simulink model "LCK_DanishV01"  (R2018b)
settings: Solver=FixedStepDiscrete  StartTime=0.0  StopTime=inf  FixedStep=0.01  RelTol=1e-3
PostLoadFcn:
  | if any(exist('dsrtsu_mdlpostloadfcn', 'file') ~= 0), dsrtsu_mdlpostloadfcn('Execute', bdroot); end
values from neighbouring files (symbols this model uses):
  C_DEG2RAD = 0.0175    [LCK_Macro.sldd]
  C_KPH2MPS = 0.2778    [LCK_Macro.sldd]
  C_NEARZERO = 0.0001    [LCK_Macro.sldd]
  C_ONE = 1.0    [LCK_Macro.sldd]
  C_RAD2DEG = 57.2958    [LCK_Macro.sldd]
  C_ZERO = 0.0    [LCK_Macro.sldd]
  k_accel_pedal_pos_per_speed_x : value not decoded    [LCK_LogicPara.sldd]
  k_accel_pedal_pos_per_speed_z : value not decoded    [LCK_LogicPara.sldd]
  k_brake_suprress_hold = 1000.0    [LCK_LogicPara.sldd]
  k_driver_appl_torque_filt = 50.0    [LCK_LogicPara.sldd]
  k_driver_suppression_hold_time = 3000.0    [LCK_LogicPara.sldd]
  k_hands_on_wheel_hold_msec = 500.0    [LCK_LogicPara.sldd]
  k_hands_on_wheel_torque_hi = 0.2    [LCK_LogicPara.sldd]
  k_hands_on_wheel_torque_lo = 0.15    [LCK_LogicPara.sldd]
  k_handsoff_delay_cycles = 50.0    [LCK_LogicPara.sldd]
  k_handsoff_torq_Lo_CR = 0.3    [LCK_LogicPara.sldd]
  k_handson_delay_cycles = 5.0    [LCK_LogicPara.sldd]
  k_HighAccel_suppress_hold = 3000.0    [LCK_LogicPara.sldd]
  k_HLR_suprress_hold = 3000.0    [LCK_LogicPara.sldd]
  k_hs_StrAng_CR_threshold_z : value not decoded    [LCK_LogicPara.sldd]
  k_LC_Exit_Switch = 0.0    [LCK_LogicPara.sldd]
  k_LCG_Configured = 1.0    [LCK_LogicPara.sldd]
  k_LCK_A0_Rdy2Act_UseConst = 0.0    [LCK_LogicPara.sldd]
  k_LCK_A0Fac_ActSta : value not decoded    [LCK_CtrlPara.sldd]
  k_LCK_A0Fac_DrvStm : value not decoded    [LCK_CtrlPara.sldd]
  k_LCK_A0Shift_LftCurv : value not decoded    [LCK_CtrlPara.sldd]
  k_LCK_A0Shift_RgtCurv : value not decoded    [LCK_CtrlPara.sldd]
  k_LCK_A0Shift_StraLan = 0.0    [LCK_CtrlPara.sldd]
  k_LCK_A0ShiftFac_Dy_LftCurv : value not decoded    [LCK_CtrlPara.sldd]
  k_LCK_A0ShiftFac_Dy_RgtCurv : value not decoded    [LCK_CtrlPara.sldd]
  k_LCK_A0ShiftFac_Vspd : value not decoded    [LCK_CtrlPara.sldd]
  k_LCK_accel_inhibit_thold = 35.0    [LCK_LogicPara.sldd]
  k_LCK_Active2Ready_Mask = 255.0    [LCK_LogicPara.sldd]
  k_LCK_CvatRateBks : value not decoded    [LCK_CtrlPara.sldd]
  k_LCK_CvatrBks : value not decoded    [LCK_CtrlPara.sldd]
  k_LCK_DFac_Dy : value not decoded    [LCK_CtrlPara.sldd]
  k_LCK_DFac_Dy_Curv : value not decoded    [LCK_CtrlPara.sldd]
  k_LCK_DFac_HaCurCen : value not decoded    [LCK_CtrlPara.sldd]
  k_LCK_DFac_HaCurSid : value not decoded    [LCK_CtrlPara.sldd]
  k_LCK_DFac_HadCurCen : value not decoded    [LCK_CtrlPara.sldd]
  k_LCK_DFac_HadCurSid : value not decoded    [LCK_CtrlPara.sldd]
  k_LCK_DFac_HadStrCen : value not decoded    [LCK_CtrlPara.sldd]
  k_LCK_DFac_HadStrSid : value not decoded    [LCK_CtrlPara.sldd]
  k_LCK_DFac_HaStrCen : value not decoded    [LCK_CtrlPara.sldd]
  k_LCK_DFac_HaStrSid : value not decoded    [LCK_CtrlPara.sldd]
  k_LCK_DFac_Rad : value not decoded    [LCK_CtrlPara.sldd]
  k_LCK_DFac_SA_CurCen : value not decoded    [LCK_CtrlPara.sldd]
  k_LCK_DFac_SA_CurSid : value not decoded    [LCK_CtrlPara.sldd]
  k_LCK_DFac_SA_StrCen : value not decoded    [LCK_CtrlPara.sldd]
  k_LCK_DFac_SA_StrSid : value not decoded    [LCK_CtrlPara.sldd]
  k_LCK_DFac_SS_CurCen : value not decoded    [LCK_CtrlPara.sldd]
  k_LCK_DFac_SS_CurSid : value not decoded    [LCK_CtrlPara.sldd]
  k_LCK_DFac_SS_StrCen : value not decoded    [LCK_CtrlPara.sldd]
  k_LCK_DFac_SS_StrSid : value not decoded    [LCK_CtrlPara.sldd]
  k_LCK_DFac_Vspd : value not decoded    [LCK_CtrlPara.sldd]
  k_LCK_DlyTm_DrvStim = 0.2    [LCK_CtrlPara.sldd]
  k_LCK_DTermMax = 2.0    [LCK_CtrlPara.sldd]
  k_LCK_DyBks_Curv : value not decoded    [LCK_CtrlPara.sldd]
  k_LCK_Enable_POOnly = 1.0    [LCK_LogicPara.sldd]
  k_LCK_Entry_DistBuffer = 0.1    [LCK_LogicPara.sldd]
  k_LCK_Fac_Vspd2RngThr_FalRec = 0.23    [LCK_CtrlPara.sldd]
  k_LCK_Ffw_CvatSwh = 0.0    [LCK_CtrlPara.sldd]
  k_LCK_Ffw_DyBks : value not decoded    [LCK_CtrlPara.sldd]
  k_LCK_Ffw_TimCon_CmdFlt = 0.0    [LCK_CtrlPara.sldd]
  k_LCK_FfwDeltaFac_Rad_Lft : value not decoded    [LCK_CtrlPara.sldd]
  k_LCK_FfwDeltaFac_Rad_Rgt : value not decoded    [LCK_CtrlPara.sldd]
  k_LCK_FfwDeltaFac_Vspd : value not decoded    [LCK_CtrlPara.sldd]
  k_LCK_FfwFac_CvatRate_Lft : value not decoded    [LCK_CtrlPara.sldd]
  k_LCK_FfwFac_CvatRate_Rgt : value not decoded    [LCK_CtrlPara.sldd]
  k_LCK_FfwFac_Dy : value not decoded    [LCK_CtrlPara.sldd]
  k_LCK_FfwFac_Rad_Lft : value not decoded    [LCK_CtrlPara.sldd]
  k_LCK_FfwFac_Rad_Rgt : value not decoded    [LCK_CtrlPara.sldd]
  k_LCK_FfwFac_Vspd : value not decoded    [LCK_CtrlPara.sldd]
  k_LCK_FfwTorq_Cvat : value not decoded    [LCK_CtrlPara.sldd]
  k_LCK_HAFac_ActSta : value not decoded    [LCK_CtrlPara.sldd]
  k_LCK_HAFac_DrvStm : value not decoded    [LCK_CtrlPara.sldd]
  k_LCK_HaloTime = 2000.0    [LCK_LogicPara.sldd]
  k_LCK_HaloTime_Switch = 0.0    [LCK_LogicPara.sldd]
  k_LCK_HARFac_ActSta : value not decoded    [LCK_CtrlPara.sldd]
  k_LCK_HARFac_DrvStm : value not decoded    [LCK_CtrlPara.sldd]
  k_LCK_Hed_DyBks : value not decoded    [LCK_CtrlPara.sldd]
  k_LCK_HedAngDiffX : value not decoded    [LCK_CtrlPara.sldd]
  k_LCK_HedAngRateDiffX : value not decoded    [LCK_CtrlPara.sldd]
  k_LCK_HndsOnWhel_DlyTm_Idl2Rdy = 0.0    [LCK_LogicPara.sldd]
  k_LCK_host_veh_width = 1.86    [LCK_LogicPara.sldd]
  k_LCK_Idle2Ready_Mask = 239.0    [LCK_LogicPara.sldd]
  k_LCK_Junc_SusTime = 1.0    [LCK_LogicPara.sldd]
  k_LCK_KpKdDecSlopeLmt = 10.0    [LCK_CtrlPara.sldd]
  k_LCK_KpKdIncSlopeLmt = 5.0    [LCK_CtrlPara.sldd]
  k_LCK_Lat_Ctrl_DFac_Lft = 1.0    [LCK_CtrlPara.sldd]
  k_LCK_Lat_Ctrl_DFac_Rgt = 1.05    [LCK_CtrlPara.sldd]
  k_LCK_Lat_Ctrl_Kd = 0.8    [LCK_CtrlPara.sldd]
  k_LCK_Lat_Ctrl_Ki = 0.5    [LCK_CtrlPara.sldd]
  k_LCK_Lat_Ctrl_Kp = 0.7    [LCK_CtrlPara.sldd]
  k_LCK_Lat_Ctrl_Kp_NearGain = 0.7    [LCK_CtrlPara.sldd]
  k_LCK_Lat_Ctrl_PFac_Lft = 1.0    [LCK_CtrlPara.sldd]
  k_LCK_Lat_Ctrl_PFac_Rgt = 1.05    [LCK_CtrlPara.sldd]
  k_LCK_Lat_Ctrl_TimCon_CmdFlt = 5.0    [LCK_CtrlPara.sldd]
  k_LCK_Lat_DFac_Rad : value not decoded    [LCK_CtrlPara.sldd]
  k_LCK_Lat_DFac_SS_Cur : value not decoded    [LCK_CtrlPara.sldd]
  k_LCK_Lat_DFac_SS_Str : value not decoded    [LCK_CtrlPara.sldd]
  k_LCK_Lat_DFac_Vspd : value not decoded    [LCK_CtrlPara.sldd]
  k_LCK_Lat_DyBks : value not decoded    [LCK_CtrlPara.sldd]
  k_LCK_Lat_IFac_Rad : value not decoded    [LCK_CtrlPara.sldd]
  k_LCK_Lat_IFac_Vspd : value not decoded    [LCK_CtrlPara.sldd]
  k_LCK_Lat_ILmtFac_Dy_CurvLan : value not decoded    [LCK_CtrlPara.sldd]
  k_LCK_Lat_ILmtFac_Dy_StraLan : value not decoded    [LCK_CtrlPara.sldd]
  k_LCK_Lat_ILmtFac_Rad : value not decoded    [LCK_CtrlPara.sldd]
  k_LCK_Lat_ILmtFac_Rad_NearGain = 1.0    [LCK_CtrlPara.sldd]
  k_LCK_Lat_ILmtFac_Vspd_CurvLan : value not decoded    [LCK_CtrlPara.sldd]
  k_LCK_Lat_ILmtFac_Vspd_StraLan : value not decoded    [LCK_CtrlPara.sldd]
  k_LCK_Lat_ITermLmt_Dy = 1.0    [LCK_CtrlPara.sldd]
  k_LCK_Lat_KpKdDecSlopeLmt = 10.0    [LCK_CtrlPara.sldd]
  k_LCK_Lat_KpKdIncSlopeLmt = 10.0    [LCK_CtrlPara.sldd]
  k_LCK_Lat_PFac_Dy_InnLftCur : value not decoded    [LCK_CtrlPara.sldd]
  k_LCK_Lat_PFac_Dy_InnRgtCur : value not decoded    [LCK_CtrlPara.sldd]
  k_LCK_Lat_PFac_Dy_OutLftCur : value not decoded    [LCK_CtrlPara.sldd]
  k_LCK_Lat_PFac_Dy_OutRgtCur : value not decoded    [LCK_CtrlPara.sldd]
  k_LCK_Lat_PFac_Dy_Str : value not decoded    [LCK_CtrlPara.sldd]
  k_LCK_Lat_PFac_Rad : value not decoded    [LCK_CtrlPara.sldd]
  ... (+153 more)
undefined symbols (not defined in the file or in its folder): k_LCK_CurvBks, K_LCK_SPA0A1A2_LMRngCmp_y
libraries: LateralControl_fcns_lib x58, simulink x24
(part 6 of 47)

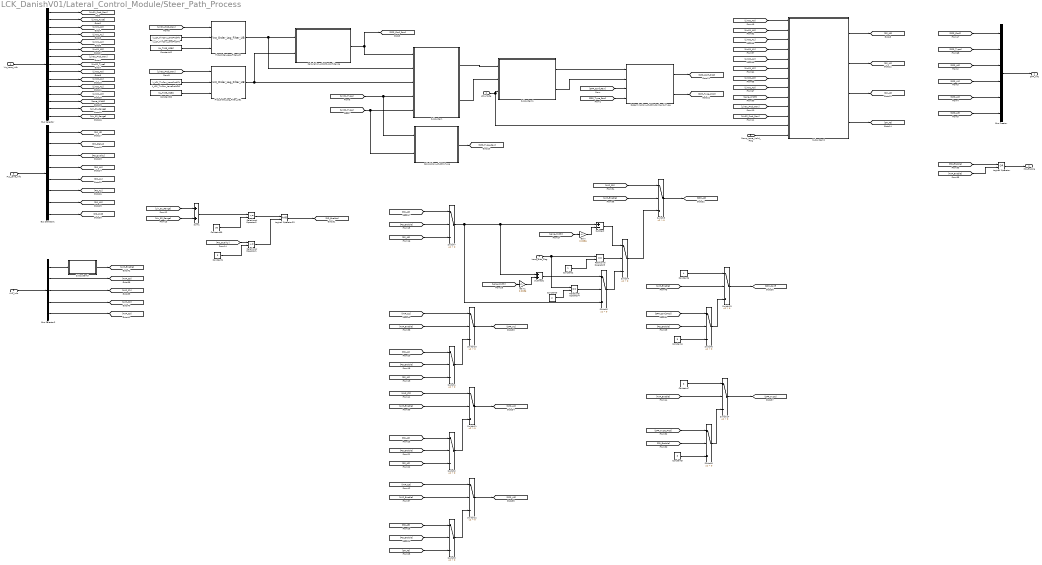
== system LCK_DanishV01/Lateral_Control_Module/Steer_Path_Process ==
  Vis_Lane_Info : Inport  Description=_GWMH9P3.Latctrl.000_23_
  LCK_Mode : Inport  Description=_GWMH9P3.Latctrl.000_23_  Port=2
  Fus_Lane_Info : Inport  Description=_GWMH9P3.Latctrl.000_23_  Port=3
  Lane_Bias_Flag : Inport  Port=4
  Ramp_Lane_Valid_Flag : Inport  Port=5
  AVP_Info : Inport  Port=6  OutDataTypeStr=Bus: AVP_OUTPUT_ST  BusOutputAsStruct=on
  Bus Creator : BusCreator  Inputs=6  OutDataTypeStr=Bus: LatCtrl_LCK_SPPInfo_t
      settings: InheritFromInputs=off
  Bus Selector : BusSelector  OutputSignals=VID_Lin_01_ProbExists,VID_Lin_01_Type,VID_Lin_01_A0,VID_Lin_01_A1,VID_Lin_01_A2,VID_Lin_01_A3,VID_Lin_02_ProbExists,VID_Lin_02_Type,VID_Lin_02_A0,VID_Lin_02_A1,VID_Lin_02_A2,VID_Lin_02_A3,VID_Lane_Width,VID_Lin_01_Range,VID_Lin_02_Range
  Bus Selector1 : BusSelector  OutputSignals=primaryObjTrajectory.id,primaryObjTrajectory.traceStatus,primaryObjTrajectory.quality,primaryObjTrajectory.curveFunc.latDistanceZeroOrderCoeff,primaryObjTrajectory.curveFunc.latDistanceFirstOrderCoeff,primaryObjTrajectory.curveFunc.latDistanceSecondOrderCoeff,primaryObjTrajectory.curveFunc.latDistanceThirdOrderCoeff,primaryObjTrajectory.curveFunc.longDistanceToend
  Bus Selector2 : BusSelector  OutputSignals=AVP_STATE,Tractory_c0,Tractory_c1,Tractory_c2,Tractory_c3
  Calculation_of_SPP_Confidence : Subsystem
  Calculation_of_SPP_Type : Subsystem
  Constant{1,4..5,7} (4 alike) : Constant  Value=3
  Constant2 : Constant
  Constant3 : Constant  Value=2
  Constant30 : Constant  Tag={'output',{'name','$P','class','EXTERN_MACRO','type','ESR_Typedefs/unsigned8_T'},'date',737462.69417376153}  Description=_GWMH9P4.LCK.000_202_  Value=ML_TIME_MSEC
  Constant42 : Constant  Tag={'output',{'name','$P','class','EXTERN_MACRO','type','ESR_Typedefs/unsigned8_T'},'date',737462.69417376153}  Description=_GWMH9P4.LCK.000_202_  Value=ML_TIME_MSEC
  Constant59 : Constant  Value=30
  Constant6 : Constant  Value=4
  Determination_of_SPP_Conf_and_Type : Subsystem
  First_Order_Lag_Filter_LIB : LateralControl_fcns_lib/First_Order_Lag_Filter_LIB  SystemSampleTime=-1
  First_Order_Lag_Filter_LIB1 : LateralControl_fcns_lib/First_Order_Lag_Filter_LIB  SystemSampleTime=-1
  Gain : Gain  Gain=0.0086
  Gain1 : Gain  Gain=0.0086
  Logical Operator : Logic  Operator=OR  AllPortsSameDT=off  OutDataTypeStr=boolean
  Logical Operator23 : Logic  AllPortsSameDT=off  OutDataTypeStr=boolean
  Relational Operator1 : RelationalOperator  OutDataTypeStr=boolean  RndMeth=Simplest
  Relational Operator2 : RelationalOperator  Operator=<=  OutDataTypeStr=boolean  RndMeth=Simplest
  Relational Operator3 : RelationalOperator  Operator===  OutDataTypeStr=boolean  RndMeth=Simplest
  Relational Operator4 : RelationalOperator  Operator===  OutDataTypeStr=boolean  RndMeth=Simplest
  Subsystem : Subsystem
  Subsystem1 : Subsystem
  Subsystem2 : Subsystem
  Subsystem3 : Subsystem
  Subtract : Sum  Inputs=+-
  Subtract1 : Sum
  Sum1 : Sum  Description=_GWMAB30P2.LCK.000_1362_  LockScale=on
  Switch{1..5,7,9..12} (10 alike) : Switch  Criteria=u2 > Threshold
  Switch{6,8,13..14} (4 alike) : Switch  Criteria=u2 > Threshold  OutDataTypeStr=single
  k_LCK_TinCon_LaneProbFlt : Constant  Tag={'output',{'name','$P','class','EXTERN_MACRO','type','ESR_Typedefs/unsigned8_T'},'date',737462.69417376153}  Description=_GWMH9P4.LCK.000_202_  Value=k_LCK_TinCon_LaneProbFlt
  k_LCK_TinCon_LaneProbFlt1 : Constant  Tag={'output',{'name','$P','class','EXTERN_MACRO','type','ESR_Typedefs/unsigned8_T'},'date',737462.69417376153}  Description=_GWMH9P4.LCK.000_202_  Value=k_LCK_TinCon_LaneProbFlt
  SPP_Info : Outport
  PO_Enable : Outport  Port=2
  wires:
  Bus Selector/5 -> [Lin01_A2]  "<VID_Lin_01_A2>"
  Constant7/1 -> Switch14/1
  [AVP_Enable] -> Switch14/2
  Switch6/1 -> Switch13/3
  Constant6/1 -> Switch13/1
  [SP_A2] -> Switch2/3
  [Lin_01_Range] -> Sum1/1
  Subsystem1/1(Lin01_Invalid) -> Determination_of_SPP_Conf_and_Type/1(Lin01_Invalid)
  Switch10/1 -> [SPP_A1]
  [AVP_Enable] -> Switch13/2
  [AVP_Enable] -> Switch9/2
  [Lin02_Type] -> Calculation_of_SPP_Type/2(Lin02_Type), Subsystem/5(Lin02_Type)
  [SPP_Type] -> Bus Creator/2  "SPP_Type"
  AVP_Info/1 -> Bus Selector2/1
  Bus Selector/9 -> [Lin02_A0]  "<VID_Lin_02_A0>"
  Calculation_of_SPP_Type/1(SPP_Type_Raw) -> [SPP_Type_Raw]
  Bus Selector/2 -> [Lin01_Type]  "<VID_Lin_01_Type>"
  [AVP_C0] -> Switch9/1
  [PO_A2] -> Switch2/1
  Subsystem/1(Lin01_ExistProb_Low) -> Subsystem1/1(Lin01_ExistProb_Low)
  [AVP_Enable] -> Switch10/2
  Bus Selector/12 -> [Lin02_A3]  "<VID_Lin_02_A3>"
  Switch14/1 -> [SPP_Type]
  [PO_A1] -> Switch1/1
  Switch2/1 -> Switch11/3
  [AVP_C3] -> Switch12/1
  Gain/1 -> Subtract/2
  Bus Creator/1 -> SPP_Info/1
  Bus Selector1/5 -> [PO_A1]  "<latDistanceFirstOrderCoeff>"
  [AVP_Enable] -> Switch11/2
  Switch9/1 -> [SPP_A0]
  Constant2/1 -> Relational Operator3/2
  Bus Selector2/3 -> [AVP_C1]  "<Tractory_c1>"
  Gain1/1 -> Subtract1/2
  Switch11/1 -> [SPP_A2]
  [SPP_Conf_Raw] -> Determination_of_SPP_Conf_and_Type/3(SPP_Conf_Raw)
  [PO_A3] -> Switch3/1
  Bus Selector2/2 -> [AVP_C0]  "<Tractory_c0>"
  Switch4/1 -> Switch9/3
  [Lane_Width] -> Subsystem2/9(Lane_Width)
  Switch1/1 -> Switch10/3
  [PO_Quality] -> Relational Operator1/1
  Constant5/1 -> Switch8/3
  Bus Selector2/1 -> Subsystem3/1(AVP_State)  "<AVP_STATE>"
  [AVP_C1] -> Switch10/1
  [PO_Enable] -> Switch7/2
  [Lane_Width] -> Gain1/1
  Switch13/1 -> [SPP_Conf]
  [Lin02_A2] -> Subsystem2/5(Lin02_A2)
  LCK_Mode/1 -> Subsystem1/3(LCK_Mode), Subsystem2/12(LCK_Mode)
  Logical Operator/1 -> PO_Enable/1
  Sum1/1 -> Relational Operator2/1
  Bus Selector2/5 -> [AVP_C3]  "<Tractory_c3>"
  Switch8/1 -> Switch14/3
  [SPP_A3] -> Bus Creator/6  "SPP_A3"
  Ramp_Lane_Valid_Flag/1 -> Subsystem2/13(Ramp_Lane_Valid_Flag)
  [AVP_Enable] -> Logical Operator/2
  [Lin01_A1] -> Subsystem2/4(Lin01_A1)
  [Lin_02_Range] -> Sum1/2
  Subsystem3/1(AVP_Enable) -> [AVP_Enable]
  Subsystem/2(Lin02_ExistProb_Low) -> Subsystem1/2(Lin02_ExistProb_Low)
  [PO_Enable] -> Switch6/2
  [PO_Enable] -> Switch8/2
  Bus Selector1/3 -> [PO_Quality]  "<quality>"
  [SPP_Conf_Prcd] -> Switch6/1
  k_LCK_TinCon_LaneProbFlt/1 -> First_Order_Lag_Filter_LIB/2
  First_Order_Lag_Filter_LIB/1 -> Calculation_of_SPP_Confidence/1(Lin01_Prob_Fltd), Subsystem/2(Lin01_Prob_Fltd)
  Constant1/1 -> Relational Operator1/2
  Constant4/1 -> Switch6/3
  [AVP_Enable] -> Switch12/2
  Constant3/1 -> Relational Operator4/2
  [Lin01_A2] -> Subsystem2/6(Lin01_A2)
  Relational Operator3/1 -> Switch4/2
  Subtract/1 -> Switch4/1
  Bus Selector2/4 -> [AVP_C2]  "<Tractory_c2>"
  [SP_A1] -> Switch1/3
  Logical Operator23/1 -> [PO_Enable]
  Subsystem2/4(SPP_A3) -> [SP_A3]
  Constant59/1 -> Relational Operator2/2
  Lane_Bias_Flag/1 -> Relational Operator4/1, Relational Operator3/1
  Subsystem2/3(SPP_A2) -> [SP_A2]
  [PO_Enable] -> Switch2/2
  Bus Selector1/6 -> [PO_A2]  "<latDistanceSecondOrderCoeff>"
  [PO_A0] -> Switch7/1
  Bus Selector1/1 -> [PO_ID]  "<id>"
  [Lin02_Prob_Raw] -> Subsystem2/11(Lin02_Prob_Fltd)
  [SPP_A2] -> Bus Creator/5  "SPP_A2"
  Fus_Lane_Info/1 -> Bus Selector1/1
  First_Order_Lag_Filter_LIB1/1 -> Subsystem/3(Lin02_Prob_Fltd), Calculation_of_SPP_Confidence/2(Lin02_Prob_Fltd)
  [Lin01_Prob_Raw] -> Subsystem2/10(Lin01_Prob_Fltd)
  [Lin01_Type] -> Calculation_of_SPP_Type/1(Lin01_Type), Subsystem/4(Lin01_Type)
  Switch3/1 -> Switch12/3
  Bus Selector/15 -> [Lin_02_Range]  "<VID_Lin_02_Range>"
  Bus Selector/6 -> [Lin01_A3]  "<VID_Lin_01_A3>"
  Bus Selector1/2 -> [PO_Status]  "<traceStatus>"
  Determination_of_SPP_Conf_and_Type/1(SPP_Conf) -> [SPP_Conf_Prcd]
  Subsystem1/2(Lin02_Invalid) -> Determination_of_SPP_Conf_and_Type/2(Lin02_Invalid)
  [Lane_Width] -> Gain/1
  Subsystem2/1(SPP_A0) -> [SP_A0]
  [PO_Enable] -> Switch1/2
  Constant30/1 -> First_Order_Lag_Filter_LIB1/3
  Bus Selector1/7 -> [PO_A3]  "<latDistanceThirdOrderCoeff>"
  [SPP_Conf] -> Bus Creator/1  "SPP_Conf"
  [Lin02_Prob_Raw] -> First_Order_Lag_Filter_LIB1/1
  Calculation_of_SPP_Confidence/1(SPP_Conf_Raw) -> [SPP_Conf_Raw], Subsystem/1(SPP_Conf_Raw)
  [SPP_Type_Prcd] -> Switch8/1
  [Lin01_Prob_Raw] -> First_Order_Lag_Filter_LIB/1
  Determination_of_SPP_Conf_and_Type/2(SPP_Type) -> [SPP_Type_Prcd]
  Relational Operator2/1 -> Logical Operator23/1
  [SP_A0] -> Switch7/3
  [SPP_A1] -> Bus Creator/4  "SPP_A1"
  [Lin02_A0] -> Subsystem2/1(Lin02_A0)
  [Lin01_A0] -> Subsystem2/2(Lin01_A0)
  Constant42/1 -> First_Order_Lag_Filter_LIB/3
  Relational Operator1/1 -> Logical Operator23/2
  [SPP_Type_Raw] -> Determination_of_SPP_Conf_and_Type/4(SPP_Type_Raw)
  k_LCK_TinCon_LaneProbFlt1/1 -> First_Order_Lag_Filter_LIB1/2
  Bus Selector/13 -> [Lane_Width]  "<VID_Lane_Width>"
  Bus Selector1/8 -> [PO_Dist]  "<longDistanceToend>"
  [SPP_A0] -> Bus Creator/3  "SPP_A0"
  [AVP_C2] -> Switch11/1
  [Lin01_A3] -> Subsystem2/8(Lin01_A3)
  Bus Selector/14 -> [Lin_01_Range]  "<VID_Lin_01_Range>"
  Subsystem2/2(SPP_A1) -> [SP_A1]
  [Lin02_A3] -> Subsystem2/7(Lin02_A3)
  [Lin02_A1] -> Subsystem2/3(Lin02_A1)
  Bus Selector/10 -> [Lin02_A1]  "<VID_Lin_02_A1>"
  Bus Selector/1 -> [Lin01_Prob_Raw]  "<VID_Lin_01_ProbExists>"
  [PO_Enable] -> Switch3/2
  Bus Selector/3 -> [Lin01_A0]  "<VID_Lin_01_A0>"
  Relational Operator4/1 -> Switch5/2
  Switch12/1 -> [SPP_A3]
  Bus Selector/7 -> [Lin02_Prob_Raw]  "<VID_Lin_02_ProbExists>"
  Subtract1/1 -> Switch5/1
  Bus Selector/8 -> [Lin02_Type]  "<VID_Lin_02_Type>"
  [PO_Enable] -> Logical Operator/1
  Switch7/1 -> Switch5/3, Subtract1/1, Subtract/1
  [SP_A3] -> Switch3/3
  Bus Selector/4 -> [Lin01_A1]  "<VID_Lin_01_A1>"
  Switch5/1 -> Switch4/3
  Vis_Lane_Info/1 -> Bus Selector/1
  Bus Selector/11 -> [Lin02_A2]  "<VID_Lin_02_A2>"
  Bus Selector1/4 -> [PO_A0]  "<latDistanceZeroOrderCoeff>"
